simulink model "PotHoleHDLDetector"  (R2022a)
settings: Solver=FixedStepDiscrete  StartTime=0.0  StopTime=9  RelTol=1e-3
PreLoadFcn:
  | % Straight lines between these corners left,right and top,bottom
  | %        ltc---rtc
  | %        /       \
  | %       /         \
  | %      /           \
  | %   lbc-------------rbc
  | %
  | % For the 320x180 image:
  | raster = [320,180];
  | ltc = [155, 66];
  | lbc = [  1,140];
  | rtc = [155, 66];
  | rbc = [285,179];
  | 
  | % fit to x = f(y) for convienence
  | abl = polyfit([lbc(2),ltc(2)],[lbc(1),ltc(1)],1);  % left side
  | abr = polyfit([rbc(2),rtc(2)],[rbc(1),rtc(1)],1);  % right side
  | leftxstart = max(  1, round((ltc(2):rbc(2))*abl(1)+abl(2)));
  | rightxend  = min(raster(1), round((ltc(2):rbc(2))*abr(1)+abr(2)));
  | startline  = min(ltc(2),rtc(2));
  | endline    = max(lbc(2),rbc(2));
  | % correct values to zero-based
  | leftxstart = leftxstart - 1;
  | rightxend = rightxend - 1;
  | startline = startline - 1;
  | endline = endline - 1;
  | %%%%%%%%%%%%%%%%
  | % Character ROM for OSD
  | load charROM16x16.mat
  | %%%%%%%%%%%%%%%%
  | % Fiducial Marker (square reticle)
  | load fiducialROM31x31.mat
undefined symbols (not defined in the file or in its folder): charROM16x16, fiducialROM, gray, Rec, SDTV
libraries: hdlsllib x62, simulink x18, visionhdlutilities x7, visionhdlio x2, dspvision x1, visionhdlfilter x1, visionhdlmorphops x1, visionhdlconversions x1, visionhdlanalysis x1
(part 1 of 2)
settings Model: DataTypeOverride=Off  SimulationMode=accelerator  Creator=The MathWorks, Inc.  LastModifiedBy=ragha
settings SolverCC: AlgebraicLoopSolver=TrustRegion
settings DataIOCC: SaveOutput=off  SaveTime=off  ReturnWorkspaceOutputs=off
settings OptimizationCC: BlockReduction=off  ConditionallyExecuteInputs=off  DefaultParameterBehavior=Inlined  EfficientMapNaN2IntZero=off
settings DebuggingCC: AlgebraicLoopMsg=error  SingleTaskRateTransMsg=error  IntegerOverflowMsg=none  ParameterPrecisionLossMsg=none  UnconnectedInputMsg=warning  UnconnectedOutputMsg=warning  UnconnectedLineMsg=warning  SFMachineParentedDataDiag=warning  IntegerSaturationMsg=none  ArithmeticOperatorsInVariantConditions=warning
settings HardwareCC: ProdBitPerPointer=32  ProdBitPerSizeT=32  ProdBitPerPtrDiffT=32  ProdLargestAtomicFloat=None  ProdIntDivRoundTo=Undefined  ProdEndianess=Unspecified  ProdWordSize=32  ProdHWDeviceType=ASIC/FPGA->ASIC/FPGA  TargetBitPerPointer=64  TargetBitPerSizeT=64  TargetBitPerPtrDiffT=64  TargetLongLongMode=on  TargetIntDivRoundTo=Zero  TargetEndianess=LittleEndian  TargetWordSize=64  TargetHWDeviceType=MATLAB Host  ProdEqTarget=off
settings SFSimCC: SimUseLocalCustomCode=off
settings RTWCC: RTWUseLocalCustomCode=off  DLArmComputeVersion=19.05
settings CodeAppCC: MaxIdLength=128
settings GRTTargetCC: TargetLangStandard=C89/C90 (ANSI)  CombineOutputUpdateFcns=off  GRTInterface=on

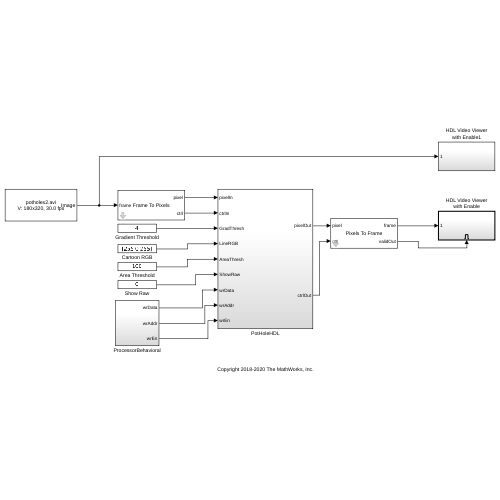
[thumbnail: Simulink's stored preview of the top-level diagram]
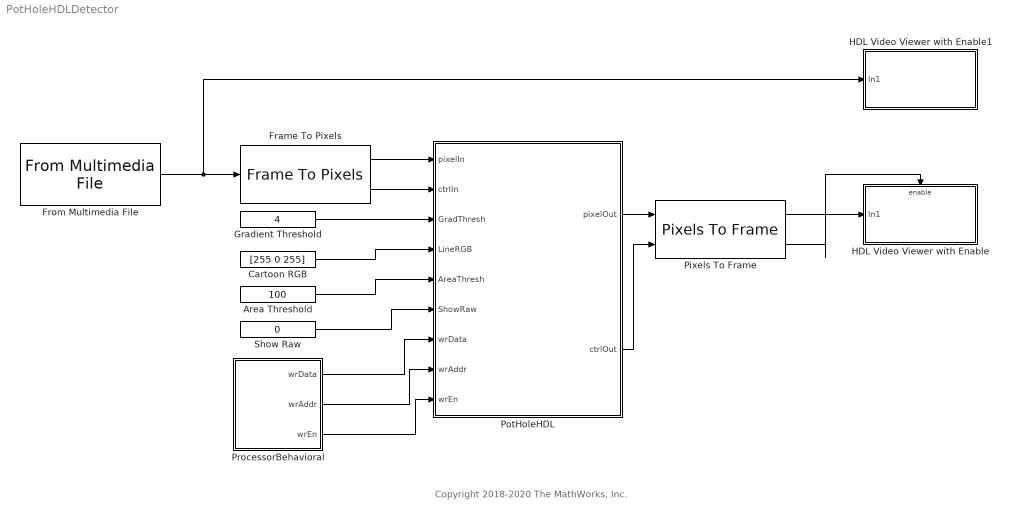
== system PotHoleHDLDetector ==
  note: Copyright 2018-2020 The MathWorks, Inc.
  "Area Threshold " : Constant  Value=100  OutDataTypeStr=fixdt(0,10,0)  SampleTime=-1
  Cartoon RGB : Constant  Value=[255 0 255]  OutDataTypeStr=uint8  SampleTime=-1
  Frame To Pixels : visionhdlio/Frame To Pixels  NumComponents=3  NumPixels=1  VideoFormat=Custom  ActivePixelsPerLine=320  ActiveVideoLines=180  TotalPixelsPerLine=400  TotalVideoLines=240  StartingActiveLine=6  FrontPorch=10  SampleTime=0  VideoFormatCache=Custom  ActivePixelsPerLineCache=320  ActiveVideoLinesCache=180  TotalPixelsPerLineCache=400  TotalVideoLinesCache=240  StartingActiveLineCache=6  FrontPorchCache=10
      settings: SourceProductBaseCode=VT
  From Multimedia File : dspvision/From Multimedia File  inputFilename=potholes2.avi  readRange=[1 Inf]  loop=on  numPlays=inf  outputStreams=Video only  videoDataType=uint8  audioDataType=int16  inheritSampleTime=on  userDefinedSampleTime=1/30  noAudioOutput=off  isIntensityVideo=off  fourcc=RGB  colorVideoFormat=One multidimensional signal  outputEOF=off  dataOrg=Column-major  audioFrameSize=1024  computeAudioFrameSize=off  outSamplingMode=Sample based
  Gradient Threshold : Constant  Value=4  OutDataTypeStr=uint8  SampleTime=-1
  HDL Video Viewer with Enable : Subsystem
  HDL Video Viewer with Enable1 : Subsystem
  Pixels To Frame : visionhdlio/Pixels To Frame  NumComponents=3  NumPixels=1  VideoFormat=Custom  ActivePixelsPerLine=320  ActiveVideoLines=180  TotalPixelsPerLine=400  TotalVideoLines=240  VideoFormatCache=Custom  ActivePixelsPerLineCache=320  ActiveVideoLinesCache=180  TotalPixelsPerLineCache=400  TotalVideoLinesCache=240
      settings: SourceProductBaseCode=VT
  PotHoleHDL : Subsystem
  ProcessorBehavioral : Subsystem
  Show Raw : Constant  Value=0  OutDataTypeStr=boolean  SampleTime=-1
  wires:
  Gradient Threshold/1 -> PotHoleHDL/3(GradThresh)
  Pixels To Frame/2 -> HDL Video Viewer with Enable/Enable
  Pixels To Frame/1 -> HDL Video Viewer with Enable/1(In1)
  PotHoleHDL/1(pixelOut) -> Pixels To Frame/1
  From Multimedia File/1 -> HDL Video Viewer with Enable1/1(In1), Frame To Pixels/1
  Cartoon RGB/1 -> PotHoleHDL/4(LineRGB)
  Frame To Pixels/2 -> PotHoleHDL/2(ctrlIn)
  Frame To Pixels/1 -> PotHoleHDL/1(pixelIn)
  "Area Threshold "/1 -> PotHoleHDL/5(AreaThresh)
  ProcessorBehavioral/1(wrData) -> PotHoleHDL/7("wrData ")
  ProcessorBehavioral/2(wrAddr) -> PotHoleHDL/8(wrAddr)
  ProcessorBehavioral/3(wrEn) -> PotHoleHDL/9(wrEn)
  Show Raw/1 -> PotHoleHDL/6(ShowRaw)
  PotHoleHDL/2(ctrlOut) -> Pixels To Frame/2

== system PotHoleHDLDetector/HDL Video Viewer with Enable ==
  In1 : Inport
  Enable : EnablePort
  PotHoleDisplay : VideoViewer  colormapValue=gray(256)  FigPos=[1 670 1280 574.666666666667]
  wires:
  In1/1 -> PotHoleDisplay/1

== system PotHoleHDLDetector/HDL Video Viewer with Enable1 ==
  In1 : Inport
  ImageIn : VideoViewer  colormapValue=gray(256)  FigPos=[128 352 321 244]
  wires:
  In1/1 -> ImageIn/1

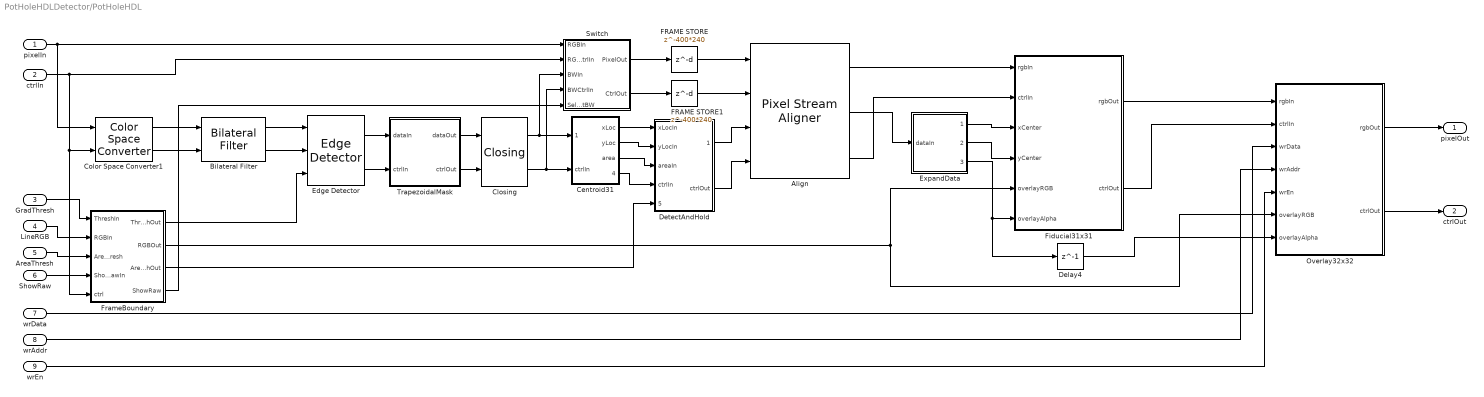
== system PotHoleHDLDetector/PotHoleHDL ==
  pixelIn : Inport
  ctrlIn : Inport  Port=2
  GradThresh : Inport  Port=3
  LineRGB : Inport  Port=4
  AreaThresh : Inport  Port=5
  ShowRaw : Inport  Port=6
  "wrData " : Inport  Port=7
  wrAddr : Inport  Port=8
  wrEn : Inport  Port=9
  Align : visionhdlutilities/Pixel Stream Aligner  LineBufferSize=2048  MaximumNumberOfLines=40  SimulateUsing=Code generation
      settings: SourceProductBaseCode=VT
  Bilateral Filter : visionhdlfilter/Bilateral Filter  NeighborhoodSize=9x9  SpatialStdDev=3  IntensityStdDev=0.75  PaddingMethod=Replicate  PaddingValue=0  LineBufferSize=2048  SimulateUsing=Code generation  CoefficientsDataTypeStr=fixdt(0,22,22)  roundingMode=Nearest  overflowMode=on  OutputDataTypeStr=fixdt(0,8,0)  OutputMin=[]  OutputMax=[]
      settings: SourceProductBaseCode=VT
  Centroid31 : Subsystem
  Closing : visionhdlmorphops/Closing  Neighborhood=[0 1 1 1 0;1 1 1 1 1;1 1 1 1 1;1 1 1 1 1;0 1 1 1 0]  LineBufferSize=2048  PaddingMethod=Constant  SimulateUsing=Code generation
      settings: SourceProductBaseCode=VT
  Color Space Converter1 : visionhdlconversions/Color Space Converter  Conversion=RGB to intensity  ConversionStandard=Rec. 601 (SDTV)  ScanningStandard=1250/50/2:1  SimulateUsing=Code generation
      settings: SourceProductBaseCode=VT
  Delay4 : Delay  DelayLength=1
  DetectAndHold : Subsystem
  Edge Detector : visionhdlanalysis/Edge Detector  Method=Sobel  BinaryImageOutputPort=on  GradientComponentOutputPorts=off  ThresholdSource=Input port  Threshold=20  LineBufferSize=2048  PaddingMethod=Symmetric  SimulateUsing=Code generation  roundingMode=Floor  overflowMode=off  GradientMin=[]  GradientMax=[]
      settings: SourceProductBaseCode=VT
  ExpandData : Subsystem
  FRAME STORE : Delay  DelayLength=400*240
  FRAME STORE1 : Delay  DelayLength=400*240
  Fiducial31x31 : Subsystem
  FrameBoundary : Subsystem
  Overlay32x32 : Subsystem
  Switch : Subsystem
  TrapezoidalMask : Subsystem
  pixelOut : Outport  VectorParamsAs1DForOutWhenUnconnected=off
  ctrlOut : Outport  Port=2  VectorParamsAs1DForOutWhenUnconnected=off
  wires:
  ctrlIn/1 -> FrameBoundary/5(ctrl), Color Space Converter1/2, Switch/2(RGBCtrlIn)
  pixelIn/1 -> Color Space Converter1/1, Switch/1(RGBIn)
  GradThresh/1 -> FrameBoundary/1(ThreshIn)
  LineRGB/1 -> FrameBoundary/2(RGBIn)
  FrameBoundary/1(ThreshOut) -> Edge Detector/3
  FrameBoundary/2(RGBOut) -> Fiducial31x31/5(overlayRGB), Overlay32x32/6(overlayRGB)
  wrEn/1 -> Overlay32x32/5(wrEn)
  Delay4/1 -> Overlay32x32/7(overlayAlpha)
  wrAddr/1 -> Overlay32x32/4(wrAddr)
  "wrData "/1 -> Overlay32x32/3(wrData)
  Overlay32x32/1(rgbOut) -> pixelOut/1
  Overlay32x32/2(ctrlOut) -> ctrlOut/1
  Closing/2 -> Switch/4(BWCtrlIn), Centroid31/2(ctrlIn)
  Color Space Converter1/1 -> Bilateral Filter/1
  Color Space Converter1/2 -> Bilateral Filter/2
  Bilateral Filter/1 -> Edge Detector/1
  Bilateral Filter/2 -> Edge Detector/2
  Edge Detector/1 -> TrapezoidalMask/1(dataIn)
  Edge Detector/2 -> TrapezoidalMask/2(ctrlIn)
  TrapezoidalMask/1(dataOut) -> Closing/1
  TrapezoidalMask/2(ctrlOut) -> Closing/2
  Closing/1 -> Switch/3(BWIn), Centroid31/1(pixelIn)
  Align/3 -> Fiducial31x31/2(ctrlIn)
  Align/1 -> Fiducial31x31/1(rgbIn)
  Fiducial31x31/2(ctrlOut) -> Overlay32x32/2(ctrlIn)
  Fiducial31x31/1(rgbOut) -> Overlay32x32/1(rgbIn)
  AreaThresh/1 -> FrameBoundary/3(AreaThresh)
  Centroid31/1(xLoc) -> DetectAndHold/1(xLocIn)
  Centroid31/2(yLoc) -> DetectAndHold/2(yLocIn)
  Centroid31/3(area) -> DetectAndHold/3(areaIn)
  FrameBoundary/3(AreaThreshOut) -> DetectAndHold/5(areaThresh)
  DetectAndHold/1(dataOut) -> Align/3
  Centroid31/4(ctrlOut) -> DetectAndHold/4(ctrlIn)
  DetectAndHold/2(ctrlOut) -> Align/4
  Align/2 -> ExpandData/1(dataIn)
  ExpandData/1(xLocOut) -> Fiducial31x31/3(xCenter)
  ExpandData/2(yLocOut) -> Fiducial31x31/4(yCenter)
  ExpandData/3(DetectOut) -> Delay4/1, Fiducial31x31/6(overlayAlpha)
  FRAME STORE/1 -> Align/1
  FRAME STORE1/1 -> Align/2
  ShowRaw/1 -> FrameBoundary/4(ShowRawIn)
  FrameBoundary/4(ShowRaw) -> Switch/5(SelectBW)
  Switch/1(PixelOut) -> FRAME STORE/1
  Switch/2(CtrlOut) -> FRAME STORE1/1

== system PotHoleHDLDetector/ProcessorBehavioral ==
  Bit Concat2 : hdlsllib/Logic and Bit Operations/Bit Concat  numInputs=2
  Constant3 : Constant  Value="uint8('     Pothole!');"
  Constant4 : Constant  Value=logical(0)
  Constant5 : Constant  Value=fi(0,0,3,0)
  Constant6 : Constant  Value=fi(0,0,2,0)
  HDL Counter2 : hdlsllib/Sources/HDL Counter  CountType=Count limited  CountInit=0  CountStep=1  CountMax=12  CountFromType=Initial value  CountFrom=0  CountResetPort=off  CountLoadPort=off  CountEnbPort=on  CountDirPort=off  CountHitOutputPort=off  CountDataType=Unsigned  CountWordLen=8  CountFracLen=0  CountSampTime=1
  Index Vector : MultiPortSwitch  DataPortOrder=Zero-based contiguous  Inputs=1  zeroidx=on  SaturateOnIntegerOverflow=off  InputSameDT=off
  Index Vector2 : MultiPortSwitch  DataPortOrder=Zero-based contiguous  Inputs=1  zeroidx=on  SaturateOnIntegerOverflow=off  InputSameDT=off
  Tapped Delay : simulink/Discrete/Tapped Delay  vinit=1  samptime=-1  NumDelays=13  DelayOrder=Oldest  includeCurrent=off
  wrData : Outport  VectorParamsAs1DForOutWhenUnconnected=off
  wrAddr : Outport  Port=2  VectorParamsAs1DForOutWhenUnconnected=off
  wrEn : Outport  Port=3  VectorParamsAs1DForOutWhenUnconnected=off
  wires:
  Tapped Delay/1 -> Index Vector/2
  Index Vector/1 -> wrEn/1, HDL Counter2/1
  Constant4/1 -> Tapped Delay/1
  Constant3/1 -> Index Vector2/2
  Index Vector2/1 -> wrData/1
  Constant6/1 -> Bit Concat2/1
  HDL Counter2/1 -> Bit Concat2/2, Index Vector2/1
  Constant5/1 -> Index Vector/1
  Bit Concat2/1 -> wrAddr/1

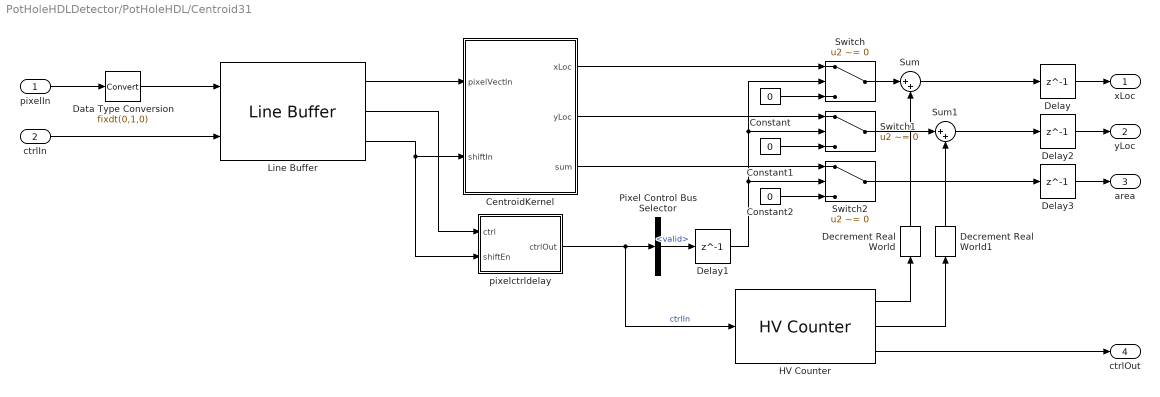
== system PotHoleHDLDetector/PotHoleHDL/Centroid31 ==
  pixelIn : Inport
  ctrlIn : Inport  Port=2
  CentroidKernel : Subsystem
  Constant : Constant  Value=0  OutDataTypeStr=Inherit: Inherit via back propagation
  Constant1 : Constant  Value=0  OutDataTypeStr=Inherit: Inherit via back propagation
  Constant2 : Constant  Value=0  OutDataTypeStr=Inherit: Inherit via back propagation
  Data Type Conversion : DataTypeConversion  OutDataTypeStr=fixdt(0,1,0)  SaturateOnIntegerOverflow=off  RndMeth=Floor
  Decrement Real World : simulink/Additional Math & Discrete/Additional Math: Increment - Decrement/Decrement Real World
      settings: SourceProductBaseCode=SL
  Decrement Real World1 : simulink/Additional Math & Discrete/Additional Math: Increment - Decrement/Decrement Real World
      settings: SourceProductBaseCode=SL
  Delay{,1..3} (4 alike) : Delay  DelayLength=1
  HV Counter : visionhdlutilities/HV Counter  ActivePixelsPerLine=320  ActiveVideoLines=180  SimulateUsing=Code generation
      settings: SourceProductBaseCode=VT
  Line Buffer : visionhdlutilities/Line Buffer  NeighborhoodSize=[31 31]  PaddingMethod=Constant  PaddingValue=0  LineBufferSize=2048  SimulateUsing=Code generation
      settings: SourceProductBaseCode=VT
  Pixel Control Bus Selector : BusSelector  OutputSignals=valid
  Sum : Sum  Inputs=|++  OutDataTypeStr=fixdt(0,11,0)  RndMeth=Convergent
  Sum1 : Sum  Inputs=|++  OutDataTypeStr=fixdt(0,11,0)  RndMeth=Convergent
  Switch : Switch  Criteria=u2 ~= 0  SaturateOnIntegerOverflow=off  InputSameDT=off
  Switch1 : Switch  Criteria=u2 ~= 0  SaturateOnIntegerOverflow=off  InputSameDT=off
  Switch2 : Switch  Criteria=u2 ~= 0  SaturateOnIntegerOverflow=off  InputSameDT=off
  pixelctrldelay : Subsystem
  xLoc : Outport  VectorParamsAs1DForOutWhenUnconnected=off
  yLoc : Outport  Port=2  VectorParamsAs1DForOutWhenUnconnected=off
  area : Outport  Port=3  VectorParamsAs1DForOutWhenUnconnected=off
  ctrlOut : Outport  Port=4  VectorParamsAs1DForOutWhenUnconnected=off
  wires:
  pixelIn/1 -> Data Type Conversion/1
  ctrlIn/1 -> Line Buffer/2
  Line Buffer/1 -> CentroidKernel/1(pixelVectIn)
  Line Buffer/3 -> pixelctrldelay/2(shiftEn), CentroidKernel/2(shiftIn)
  Data Type Conversion/1 -> Line Buffer/1
  pixelctrldelay/1(ctrlOut) -> HV Counter/1, Pixel Control Bus Selector/1  "ctrlIn"
  CentroidKernel/1(xLoc) -> Switch/1
  Switch2/1 -> Delay3/1
  CentroidKernel/2(yLoc) -> Switch1/1
  CentroidKernel/3(sum) -> Switch2/1
  Constant/1 -> Switch/3
  Constant1/1 -> Switch1/3
  Constant2/1 -> Switch2/3
  Pixel Control Bus Selector/1 -> Delay1/1  "<valid>"
  Delay/1 -> xLoc/1
  Delay2/1 -> yLoc/1
  Delay3/1 -> area/1
  Switch/1 -> Sum/1
  Sum/1 -> Delay/1
  Switch1/1 -> Sum1/1
  Sum1/1 -> Delay2/1
  Line Buffer/2 -> pixelctrldelay/1(ctrl)
  HV Counter/1 -> Decrement Real World/1
  HV Counter/2 -> Decrement Real World1/1
  HV Counter/3 -> ctrlOut/1
  Delay1/1 -> Switch2/2, Switch1/2, Switch/2
  Decrement Real World/1 -> Sum/2
  Decrement Real World1/1 -> Sum1/2

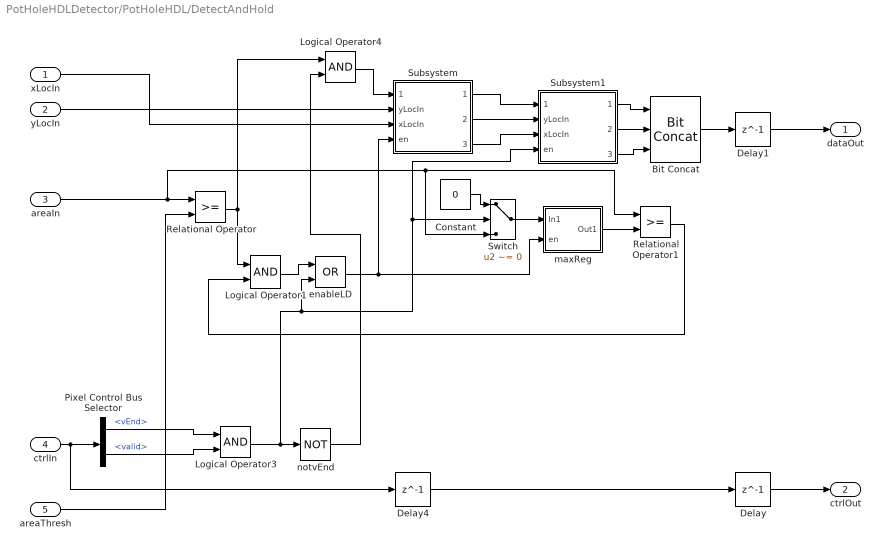
== system PotHoleHDLDetector/PotHoleHDL/DetectAndHold ==
  xLocIn : Inport
  yLocIn : Inport  Port=2
  areaIn : Inport  Port=3
  ctrlIn : Inport  Port=4
  areaThresh : Inport  Port=5
  Bit Concat : hdlsllib/Logic and Bit Operations/Bit Concat  numInputs=3
  Constant : Constant  Value=0  OutDataTypeStr=fixdt(0,10,0)
  Delay : Delay  DelayLength=1
  Delay1 : Delay  DelayLength=1
  Delay4 : Delay  DelayLength=1
  Logical Operator1 : Logic  AllPortsSameDT=off  OutDataTypeStr=boolean
  Logical Operator3 : Logic  AllPortsSameDT=off  OutDataTypeStr=boolean
  Logical Operator4 : Logic  AllPortsSameDT=off  OutDataTypeStr=boolean
  Pixel Control Bus Selector : BusSelector  OutputSignals=vEnd,valid
  Relational Operator : RelationalOperator  OutDataTypeStr=boolean  RndMeth=Simplest  InputSameDT=off
  Relational Operator1 : RelationalOperator  OutDataTypeStr=boolean  RndMeth=Simplest  InputSameDT=off
  Subsystem : Subsystem
  Subsystem1 : Subsystem
  Switch : Switch  Criteria=u2 ~= 0  SaturateOnIntegerOverflow=off  InputSameDT=off
  enableLD : Logic  Operator=OR  AllPortsSameDT=off  OutDataTypeStr=boolean
  maxReg : Subsystem
  notvEnd : Logic  Operator=NOT  AllPortsSameDT=off  OutDataTypeStr=boolean
  dataOut : Outport  VectorParamsAs1DForOutWhenUnconnected=off
  ctrlOut : Outport  Port=2  VectorParamsAs1DForOutWhenUnconnected=off
  wires:
  Logical Operator3/1 -> notvEnd/1, Subsystem1/4(en), Switch/2, enableLD/2
  areaIn/1 -> Switch/3, Relational Operator1/1, Relational Operator/1
  Pixel Control Bus Selector/1 -> Logical Operator3/1  "<vEnd>"
  Pixel Control Bus Selector/2 -> Logical Operator3/2  "<valid>"
  Relational Operator/1 -> Logical Operator4/1, Logical Operator1/1
  notvEnd/1 -> Logical Operator4/2
  ctrlIn/1 -> Pixel Control Bus Selector/1, Delay4/1
  areaThresh/1 -> Relational Operator/2
  Delay4/1 -> Delay/1
  Delay/1 -> ctrlOut/1
  Delay1/1 -> dataOut/1
  Logical Operator1/1 -> enableLD/1
  Logical Operator4/1 -> Subsystem/1(detectIn)
  maxReg/1(Out1) -> Relational Operator1/2
  enableLD/1 -> maxReg/2(en), Subsystem/4(en)
  Switch/1 -> maxReg/1(In1)
  Relational Operator1/1 -> Logical Operator1/2
  yLocIn/1 -> Subsystem/2(yLocIn)
  xLocIn/1 -> Subsystem/3(xLocIn)
  Subsystem/3(xLocOut) -> Subsystem1/3(xLocIn)
  Subsystem/2(yLocOut) -> Subsystem1/2(yLocIn)
  Subsystem/1(detectOut) -> Subsystem1/1(detectIn)
  Constant/1 -> Switch/1
  Subsystem1/2(yLocOut) -> Bit Concat/2
  Subsystem1/3(xLocOut) -> Bit Concat/3
  Subsystem1/1(detectOut) -> Bit Concat/1
  Bit Concat/1 -> Delay1/1

== system PotHoleHDLDetector/PotHoleHDL/ExpandData ==
  dataIn : Inport
  Bit Slice : hdlsllib/Logic and Bit Operations/Bit Slice  lidx=10  ridx=0
      settings: SourceProductBaseCode=SL
  Bit Slice1 : hdlsllib/Logic and Bit Operations/Bit Slice  lidx=21  ridx=11
      settings: SourceProductBaseCode=SL
  Bit Slice2 : hdlsllib/Logic and Bit Operations/Bit Slice  lidx=22  ridx=22
      settings: SourceProductBaseCode=SL
  Gain : Gain  Gain=255  ParamDataTypeStr=uint8  OutDataTypeStr=uint8
  xLocOut : Outport  VectorParamsAs1DForOutWhenUnconnected=off
  yLocOut : Outport  Port=2  VectorParamsAs1DForOutWhenUnconnected=off
  DetectOut : Outport  Port=3  VectorParamsAs1DForOutWhenUnconnected=off
  wires:
  Bit Slice2/1 -> Gain/1
  dataIn/1 -> Bit Slice2/1, Bit Slice1/1, Bit Slice/1
  Bit Slice/1 -> xLocOut/1
  Bit Slice1/1 -> yLocOut/1
  Gain/1 -> DetectOut/1

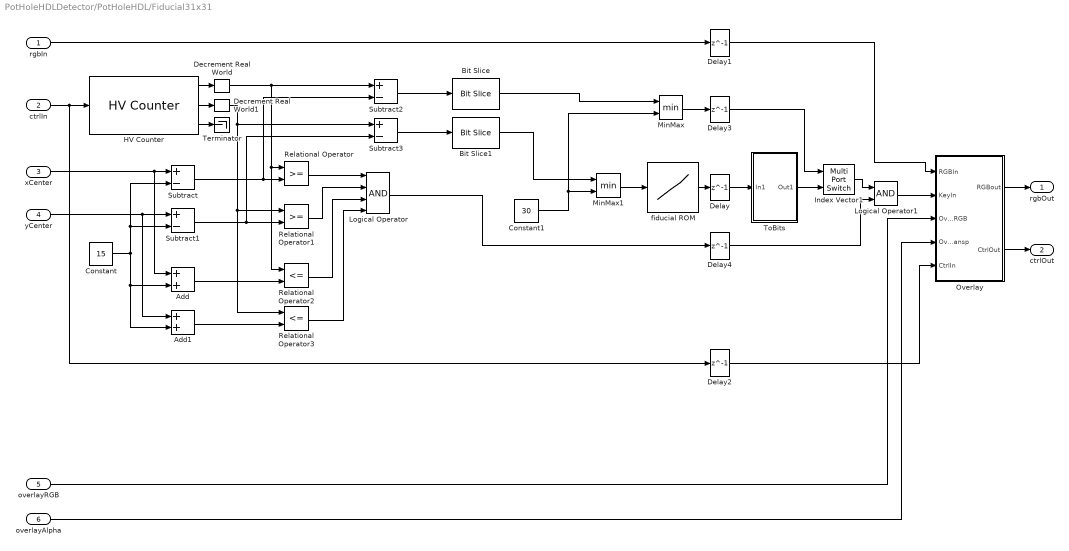
== system PotHoleHDLDetector/PotHoleHDL/Fiducial31x31 ==
  rgbIn : Inport
  ctrlIn : Inport  Port=2
  xCenter : Inport  Port=3
  yCenter : Inport  Port=4
  overlayRGB : Inport  Port=5
  overlayAlpha : Inport  Port=6
  Add : Sum
  Add1 : Sum
  Bit Slice : hdlsllib/Logic and Bit Operations/Bit Slice  lidx=4  ridx=0
      settings: SourceProductBaseCode=SL
  Bit Slice1 : hdlsllib/Logic and Bit Operations/Bit Slice  lidx=4  ridx=0
      settings: SourceProductBaseCode=SL
  Constant : Constant  Value=15  OutDataTypeStr=fixdt(0,11,0)
  Constant1 : Constant  Value=30  OutDataTypeStr=fixdt(0,5,0)
  Decrement Real World : simulink/Additional Math & Discrete/Additional Math: Increment - Decrement/Decrement Real World
      settings: SourceProductBaseCode=SL
  Decrement Real World1 : simulink/Additional Math & Discrete/Additional Math: Increment - Decrement/Decrement Real World
      settings: SourceProductBaseCode=SL
  Delay{,1..4} (5 alike) : Delay  DelayLength=1
  HV Counter : visionhdlutilities/HV Counter  ActivePixelsPerLine=1920  ActiveVideoLines=1080  SimulateUsing=Code generation
      settings: SourceProductBaseCode=VT
  Index Vector1 : MultiPortSwitch  DataPortOrder=Zero-based contiguous  Inputs=1  zeroidx=on  SaturateOnIntegerOverflow=off  InputSameDT=off
  Logical Operator : Logic  Inputs=4  AllPortsSameDT=off  OutDataTypeStr=boolean
  Logical Operator1 : Logic  AllPortsSameDT=off  OutDataTypeStr=boolean
  MinMax : MinMax  Inputs=2
  MinMax1 : MinMax  Inputs=2
  Overlay : Subsystem
  Relational Operator : RelationalOperator  OutDataTypeStr=boolean  RndMeth=Simplest  InputSameDT=off
  Relational Operator1 : RelationalOperator  OutDataTypeStr=boolean  RndMeth=Simplest  InputSameDT=off
  Relational Operator2 : RelationalOperator  Operator=<=  OutDataTypeStr=boolean  RndMeth=Simplest  InputSameDT=off
  Relational Operator3 : RelationalOperator  Operator=<=  OutDataTypeStr=boolean  RndMeth=Simplest  InputSameDT=off
  Subtract{,1..3} (4 alike) : Sum  Inputs=+-
  Terminator : Terminator
  ToBits : Subsystem
  fiducial ROM : Lookup_n-D  NumberOfTableDimensions=1  LookupTableObject=''  BreakpointsForDimension1=[0:30]  BreakpointsForDimension1FirstPoint=10  BreakpointsForDimension2FirstPoint=10  BreakpointsForDimension1Spacing=12  BreakpointsForDimension2Spacing=12  IndexSearchMethod=Evenly spaced points  Table=fiducialROM  TableDataTypeStr=fixdt(0,31,0)  InterpMethod=Flat  DiagnosticForOutOfRangeInput=Error  InternalRulePriority=Speed  OutDataTypeStr=fixdt(0,31,0)  RndMeth=Simplest
  rgbOut : Outport  VectorParamsAs1DForOutWhenUnconnected=off
  ctrlOut : Outport  Port=2  VectorParamsAs1DForOutWhenUnconnected=off
  wires:
  ctrlIn/1 -> Delay2/1, HV Counter/1
  rgbIn/1 -> Delay1/1
  Overlay/2("CtrlOut ") -> ctrlOut/1
  Decrement Real World/1 -> Relational Operator2/1, Relational Operator/1, Subtract2/1
  fiducial ROM/1 -> Delay/1
  overlayRGB/1 -> Overlay/3(OverlayRGB)
  overlayAlpha/1 -> Overlay/4(OverlayTransp)
  Delay2/1 -> Overlay/5(CtrlIn)
  Overlay/1(RGBout) -> rgbOut/1
  Delay1/1 -> Overlay/1(RGBIn)
  Delay3/1 -> Index Vector1/1
  Decrement Real World1/1 -> Subtract3/1, Relational Operator1/1, Relational Operator3/1
  xCenter/1 -> Add/1, Subtract/1
  yCenter/1 -> Add1/1, Subtract1/1
  Constant/1 -> Add/2, Add1/2, Subtract1/2, Subtract/2
  Subtract/1 -> Subtract2/2, Relational Operator/2
  Subtract1/1 -> Subtract3/2, Relational Operator1/2
  Add/1 -> Relational Operator2/2
  Add1/1 -> Relational Operator3/2
  Relational Operator/1 -> Logical Operator/1
  Relational Operator1/1 -> Logical Operator/2
  Relational Operator2/1 -> Logical Operator/3
  Relational Operator3/1 -> Logical Operator/4
  Logical Operator/1 -> Delay4/1
  Subtract2/1 -> Bit Slice/1
  Subtract3/1 -> Bit Slice1/1
  Index Vector1/1 -> Logical Operator1/1
  Delay4/1 -> Logical Operator1/2
  Bit Slice/1 -> MinMax/1
  MinMax/1 -> Delay3/1
  Constant1/1 -> MinMax1/2, MinMax/2
  MinMax1/1 -> fiducial ROM/1
  Bit Slice1/1 -> MinMax1/1
  Logical Operator1/1 -> Overlay/2(KeyIn)
  ToBits/1(Out1) -> Index Vector1/2
  Delay/1 -> ToBits/1(In1)
  HV Counter/1 -> Decrement Real World/1
  HV Counter/2 -> Decrement Real World1/1
  HV Counter/3 -> Terminator/1

== system PotHoleHDLDetector/PotHoleHDL/FrameBoundary ==
  ThreshIn : Inport
  RGBIn : Inport  Port=2
  AreaThresh : Inport  Port=3
  ShowRawIn : Inport  Port=4
  ctrl : Inport  Port=5
  Delay{,1..3} (4 alike) : Delay  DelayLength=1  ShowEnablePort=on
      settings: InputPortMap=u0,e6
  Logical Operator : Logic  AllPortsSameDT=off  OutDataTypeStr=boolean
  Pixel Control Bus Selector : BusSelector  OutputSignals=vStart,valid
  ThreshOut : Outport  VectorParamsAs1DForOutWhenUnconnected=off
  RGBOut : Outport  Port=2  VectorParamsAs1DForOutWhenUnconnected=off
  AreaThreshOut : Outport  Port=3  VectorParamsAs1DForOutWhenUnconnected=off
  ShowRaw : Outport  Port=4  VectorParamsAs1DForOutWhenUnconnected=off
  wires:
  ctrl/1 -> Pixel Control Bus Selector/1
  Pixel Control Bus Selector/1 -> Logical Operator/1  "<vStart>"
  ThreshIn/1 -> Delay/1
  Logical Operator/1 -> Delay3/2, Delay2/2, Delay1/2, Delay/2
  Pixel Control Bus Selector/2 -> Logical Operator/2  "<valid>"
  Delay1/1 -> RGBOut/1
  RGBIn/1 -> Delay1/1
  Delay/1 -> ThreshOut/1
  AreaThresh/1 -> Delay2/1
  Delay2/1 -> AreaThreshOut/1
  Delay3/1 -> ShowRaw/1
  ShowRawIn/1 -> Delay3/1

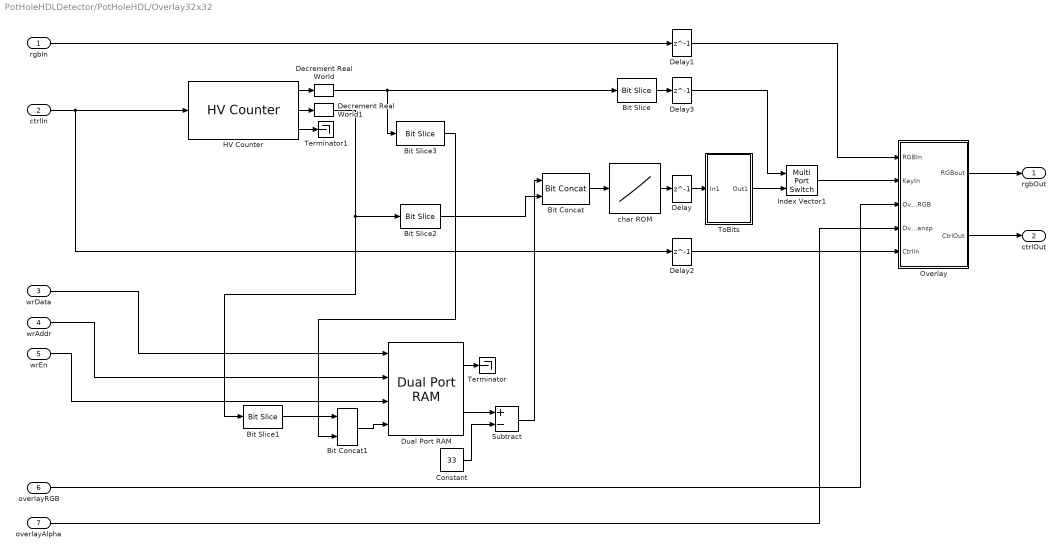
== system PotHoleHDLDetector/PotHoleHDL/Overlay32x32 ==
  rgbIn : Inport
  ctrlIn : Inport  Port=2
  wrData : Inport  Port=3
  wrAddr : Inport  Port=4
  wrEn : Inport  Port=5
  overlayRGB : Inport  Port=6
  overlayAlpha : Inport  Port=7
  Bit Concat : hdlsllib/Logic and Bit Operations/Bit Concat  numInputs=2
  Bit Concat1 : hdlsllib/Logic and Bit Operations/Bit Concat  numInputs=2
  Bit Slice : hdlsllib/Logic and Bit Operations/Bit Slice  lidx=3  ridx=0
      settings: SourceProductBaseCode=SL
  Bit Slice1 : hdlsllib/Logic and Bit Operations/Bit Slice  lidx=8  ridx=4
      settings: SourceProductBaseCode=SL
  Bit Slice2 : hdlsllib/Logic and Bit Operations/Bit Slice  lidx=3  ridx=0
      settings: SourceProductBaseCode=SL
  Bit Slice3 : hdlsllib/Logic and Bit Operations/Bit Slice  lidx=8  ridx=4
      settings: SourceProductBaseCode=SL
  Constant : Constant  Value=33  OutDataTypeStr=uint8
  Decrement Real World : simulink/Additional Math & Discrete/Additional Math: Increment - Decrement/Decrement Real World
      settings: SourceProductBaseCode=SL
  Decrement Real World1 : simulink/Additional Math & Discrete/Additional Math: Increment - Decrement/Decrement Real World
      settings: SourceProductBaseCode=SL
  Delay{,1..3} (4 alike) : Delay  DelayLength=1
  Dual Port RAM : hdlsllib/HDL RAMs/Dual Port RAM  ram_size=10
      settings: SourceProductBaseCode=SL
  HV Counter : visionhdlutilities/HV Counter  ActivePixelsPerLine=1920  ActiveVideoLines=1080  SimulateUsing=Code generation
      settings: SourceProductBaseCode=VT
  Index Vector1 : MultiPortSwitch  DataPortOrder=Zero-based contiguous  Inputs=1  zeroidx=on  SaturateOnIntegerOverflow=off  InputSameDT=off
  Overlay : Subsystem
  Subtract : Sum  Inputs=+-  OutDataTypeStr=fixdt(0,7,0)
  Terminator : Terminator
  Terminator1 : Terminator
  ToBits : Subsystem
  char ROM : Lookup_n-D  NumberOfTableDimensions=1  LookupTableObject=''  BreakpointsForDimension1=[0:128*16-1]  BreakpointsForDimension1FirstPoint=10  BreakpointsForDimension2FirstPoint=10  BreakpointsForDimension1Spacing=12  BreakpointsForDimension2Spacing=12  IndexSearchMethod=Evenly spaced points  Table=charROM16x16  TableDataTypeStr=fixdt(0,16,0)  InterpMethod=Flat  DiagnosticForOutOfRangeInput=Error  InternalRulePriority=Speed  OutDataTypeStr=fixdt(0,16,0)  RndMeth=Simplest
  rgbOut : Outport  VectorParamsAs1DForOutWhenUnconnected=off
  ctrlOut : Outport  Port=2  VectorParamsAs1DForOutWhenUnconnected=off
  wires:
  ctrlIn/1 -> Delay2/1, HV Counter/1
  rgbIn/1 -> Delay1/1
  Overlay/2("CtrlOut ") -> ctrlOut/1
  Bit Slice/1 -> Delay3/1
  ToBits/1(Out1) -> Index Vector1/2
  HV Counter/1 -> Decrement Real World/1
  Index Vector1/1 -> Overlay/2(KeyIn)
  Delay/1 -> ToBits/1(In1)
  Bit Concat/1 -> char ROM/1
  char ROM/1 -> Delay/1
  overlayRGB/1 -> Overlay/3(OverlayRGB)
  overlayAlpha/1 -> Overlay/4(OverlayTransp)
  Delay2/1 -> Overlay/5(CtrlIn)
  Overlay/1(RGBout) -> rgbOut/1
  Delay1/1 -> Overlay/1(RGBIn)
  Delay3/1 -> Index Vector1/1
  Bit Slice2/1 -> Bit Concat/2
  HV Counter/2 -> Decrement Real World1/1
  Subtract/1 -> Bit Concat/1
  Dual Port RAM/2 -> Subtract/1
  Constant/1 -> Subtract/2
  Bit Concat1/1 -> Dual Port RAM/4
  Bit Slice3/1 -> Bit Concat1/2
  Bit Slice1/1 -> Bit Concat1/1
  wrData/1 -> Dual Port RAM/1
  wrAddr/1 -> Dual Port RAM/2
  wrEn/1 -> Dual Port RAM/3
  Dual Port RAM/1 -> Terminator/1
  HV Counter/3 -> Terminator1/1
  Decrement Real World/1 -> Bit Slice3/1, Bit Slice/1
  Decrement Real World1/1 -> Bit Slice1/1, Bit Slice2/1

== system PotHoleHDLDetector/PotHoleHDL/Switch ==
  RGBIn : Inport
  RGBCtrlIn : Inport  Port=2
  BWIn : Inport  Port=3
  BWCtrlIn : Inport  Port=4
  SelectBW : Inport  Port=5
  Gain1 : Gain  Gain=255  ParamDataTypeStr=uint8  OutDataTypeStr=uint8
  Mux : Mux  Inputs=3
  Switch : Switch  Criteria=u2 ~= 0  SaturateOnIntegerOverflow=off  InputSameDT=off
  Switch1 : Switch  Criteria=u2 ~= 0  SaturateOnIntegerOverflow=off  InputSameDT=off
  PixelOut : Outport  VectorParamsAs1DForOutWhenUnconnected=off
  CtrlOut : Outport  Port=2  VectorParamsAs1DForOutWhenUnconnected=off
  wires:
  RGBCtrlIn/1 -> Switch1/3
  Gain1/1 -> Mux/3, Mux/2, Mux/1
  Mux/1 -> Switch/1
  Switch/1 -> PixelOut/1
  BWCtrlIn/1 -> Switch1/1
  SelectBW/1 -> Switch1/2, Switch/2
  RGBIn/1 -> Switch/3
  BWIn/1 -> Gain1/1
  Switch1/1 -> CtrlOut/1

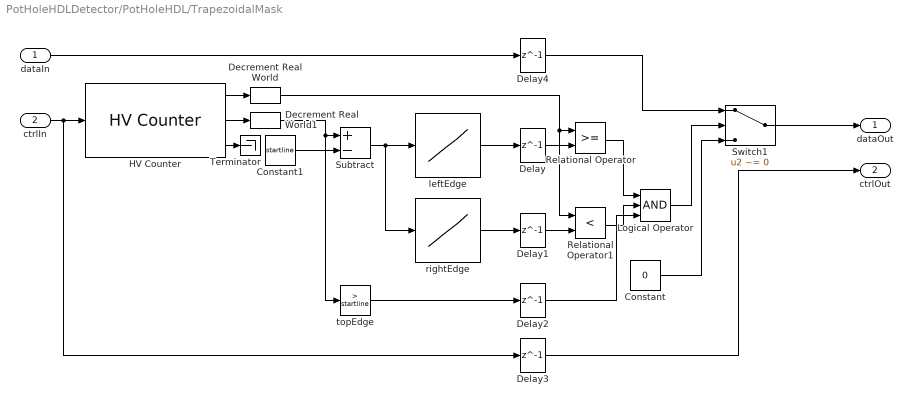
== system PotHoleHDLDetector/PotHoleHDL/TrapezoidalMask ==
  dataIn : Inport
  ctrlIn : Inport  Port=2
  Constant : Constant  Value=0  OutDataTypeStr=Inherit: Inherit via back propagation
  Constant1 : Constant  Value=startline  OutDataTypeStr=fixdt(0,11,0)
  Decrement Real World : simulink/Additional Math & Discrete/Additional Math: Increment - Decrement/Decrement Real World
      settings: SourceProductBaseCode=SL
  Decrement Real World1 : simulink/Additional Math & Discrete/Additional Math: Increment - Decrement/Decrement Real World
      settings: SourceProductBaseCode=SL
  Delay{,1..4} (5 alike) : Delay  DelayLength=1
  HV Counter : visionhdlutilities/HV Counter  ActivePixelsPerLine=320  ActiveVideoLines=240  SimulateUsing=Code generation
      settings: SourceProductBaseCode=VT
  Logical Operator : Logic  Inputs=3  AllPortsSameDT=off  OutDataTypeStr=boolean
  Relational Operator : RelationalOperator  OutDataTypeStr=boolean  RndMeth=Simplest  InputSameDT=off
  Relational Operator1 : RelationalOperator  Operator=<  OutDataTypeStr=boolean  RndMeth=Simplest  InputSameDT=off
  Subtract : Sum  Inputs=+-  OutDataTypeStr=Inherit: Same as first input
  Switch1 : Switch  Criteria=u2 ~= 0  SaturateOnIntegerOverflow=off  InputSameDT=off
  Terminator : Terminator
  leftEdge : Lookup_n-D  NumberOfTableDimensions=1  LookupTableObject=''  BreakpointsForDimension1=[0:113]  BreakpointsForDimension1FirstPoint=10  BreakpointsForDimension2FirstPoint=10  BreakpointsForDimension1Spacing=12  BreakpointsForDimension2Spacing=12  IndexSearchMethod=Evenly spaced points  Table=leftxstart  TableDataTypeStr=fixdt(0,11,0)  InterpMethod=Flat  InternalRulePriority=Speed  OutDataTypeStr=fixdt(0,11,0)  RndMeth=Simplest
  rightEdge : Lookup_n-D  NumberOfTableDimensions=1  LookupTableObject=''  BreakpointsForDimension1=[0:113]  BreakpointsForDimension1FirstPoint=10  BreakpointsForDimension2FirstPoint=10  BreakpointsForDimension1Spacing=12  BreakpointsForDimension2Spacing=12  IndexSearchMethod=Evenly spaced points  Table=rightxend  TableDataTypeStr=fixdt(0,11,0)  InterpMethod=Flat  InternalRulePriority=Speed  OutDataTypeStr=fixdt(0,11,0)  RndMeth=Simplest
  topEdge : simulink/Logic and Bit Operations/Compare To Constant  relop=>  const=startline  OutDataTypeStr=boolean
  dataOut : Outport  VectorParamsAs1DForOutWhenUnconnected=off
  ctrlOut : Outport  Port=2  VectorParamsAs1DForOutWhenUnconnected=off
  wires:
  rightEdge/1 -> Delay1/1
  topEdge/1 -> Delay2/1
  HV Counter/1 -> Decrement Real World/1
  leftEdge/1 -> Delay/1
  HV Counter/2 -> Decrement Real World1/1
  Relational Operator1/1 -> Logical Operator/2
  Logical Operator/1 -> Switch1/2
  Constant/1 -> Switch1/3
  Relational Operator/1 -> Logical Operator/1
  Delay2/1 -> Logical Operator/3
  Delay1/1 -> Relational Operator1/2
  Delay/1 -> Relational Operator/2
  dataIn/1 -> Delay4/1
  Switch1/1 -> dataOut/1
  ctrlIn/1 -> HV Counter/1, Delay3/1
  Delay3/1 -> ctrlOut/1
  Subtract/1 -> rightEdge/1, leftEdge/1
  Constant1/1 -> Subtract/2
  Delay4/1 -> Switch1/1
  HV Counter/3 -> Terminator/1
  Decrement Real World/1 -> Relational Operator1/1, Relational Operator/1
  Decrement Real World1/1 -> Subtract/1, topEdge/1

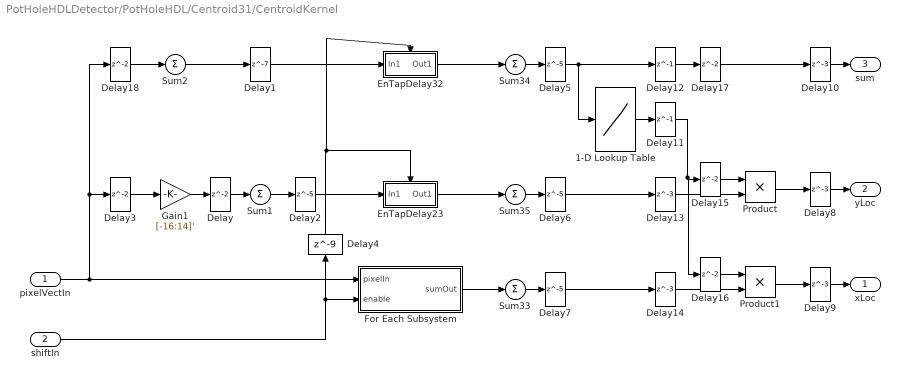
== system PotHoleHDLDetector/PotHoleHDL/Centroid31/CentroidKernel ==
  pixelVectIn : Inport
  shiftIn : Inport  Port=2
  1-D Lookup Table : Lookup_n-D  NumberOfTableDimensions=1  LookupTableObject=''  BreakpointsForDimension1=[0:1023]  BreakpointsForDimension1FirstPoint=10  BreakpointsForDimension2FirstPoint=10  BreakpointsForDimension1Spacing=12  BreakpointsForDimension2Spacing=12  IndexSearchMethod=Evenly spaced points  Table=1./[1,1:1023]  TableDataTypeStr=fixdt(0,15,15)  InterpMethod=Flat  DiagnosticForOutOfRangeInput=Error  InternalRulePriority=Speed  OutDataTypeStr=fixdt(0,15,15)  RndMeth=Simplest
  Delay{,3,15..18} (6 alike) : Delay
  Delay1 : Delay  DelayLength=7
  Delay{8..10,13..14} (5 alike) : Delay  DelayLength=3
  Delay11 : Delay  DelayLength=1
  Delay12 : Delay  DelayLength=1
  Delay{2,5..7} (4 alike) : Delay  DelayLength=5
  Delay4 : Delay  DelayLength=9
  EnTapDelay23 : Subsystem
  EnTapDelay32 : Subsystem
  For Each Subsystem : Subsystem  TreatAsAtomicUnit=on
  Gain1 : Gain  Gain=[-16:14]'  ParamDataTypeStr=fixdt(1,5,0)  OutDataTypeStr=fixdt(1,5,0)
  Product : Product  OutDataTypeStr=fixdt(1,8,3)  RndMeth=Nearest  SaturateOnIntegerOverflow=on
  Product1 : Product  OutDataTypeStr=fixdt(1,8,3)  RndMeth=Nearest  SaturateOnIntegerOverflow=on
  Sum{1..2,33..35} (5 alike) : Sum  Inputs=1
  xLoc : Outport  VectorParamsAs1DForOutWhenUnconnected=off
  yLoc : Outport  Port=2  VectorParamsAs1DForOutWhenUnconnected=off
  sum : Outport  Port=3  VectorParamsAs1DForOutWhenUnconnected=off
  wires:
  pixelVectIn/1 -> For Each Subsystem/1(pixelIn), Delay18/1, Delay3/1
  Sum1/1 -> Delay2/1
  EnTapDelay23/1(Out1) -> Sum35/1
  EnTapDelay32/1(Out1) -> Sum34/1
  Sum34/1 -> Delay5/1
  Product/1 -> Delay8/1
  Sum35/1 -> Delay6/1
  Product1/1 -> Delay9/1
  Sum33/1 -> Delay7/1
  1-D Lookup Table/1 -> Delay11/1
  shiftIn/1 -> For Each Subsystem/2(enable), Delay4/1
  For Each Subsystem/1(sumOut) -> Sum33/1
  Delay1/1 -> EnTapDelay32/1(In1)
  Delay2/1 -> EnTapDelay23/1(In1)
  Delay/1 -> Sum1/1
  Gain1/1 -> Delay/1
  Delay3/1 -> Gain1/1
  Delay4/1 -> EnTapDelay32/Enable, EnTapDelay23/Enable
  Delay5/1 -> 1-D Lookup Table/1, Delay12/1
  Delay6/1 -> Delay13/1
  Delay7/1 -> Delay14/1
  Delay8/1 -> yLoc/1
  Delay9/1 -> xLoc/1
  Delay10/1 -> sum/1
  Delay11/1 -> Delay16/1, Delay15/1
  Delay12/1 -> Delay17/1
  Delay13/1 -> Product/2
  Delay14/1 -> Product1/2
  Delay15/1 -> Product/1
  Delay16/1 -> Product1/1
  Delay17/1 -> Delay10/1
  Delay18/1 -> Sum2/1
  Sum2/1 -> Delay1/1

== system PotHoleHDLDetector/PotHoleHDL/Centroid31/pixelctrldelay ==
  ctrl : Inport
  shiftEn : Inport  Port=2
  Bitwise AND{,1..4} (5 alike) : simulink/Logic and Bit Operations/Bitwise Operator  logicop=AND  UseBitMask=off  NumInputPorts=2  BitMask=bin2dec('11011001')  BitMaskRealWorld=Stored Integer
  Delay : Delay  DelayLength=16  ShowEnablePort=on
      settings: InputPortMap=u0,e6
  Delay1 : Delay  DelayLength=1
  Delay2 : Delay  DelayLength=19
  Pixel Control Bus Creator : visionhdlutilities/Pixel Control Bus Creator
      settings: SourceProductBaseCode=VT
  Pixel Control Bus Selector : BusSelector  OutputSignals=hStart,hEnd,vStart,vEnd,valid
  State Control : StateControl  StateControl=Synchronous
  ctrlOut : Outport  VectorParamsAs1DForOutWhenUnconnected=off
  wires:
  Bitwise AND4/1 -> Pixel Control Bus Creator/5
  Bitwise AND/1 -> Pixel Control Bus Creator/1
  Pixel Control Bus Selector/3 -> Bitwise AND2/1  "<vStart>"
  Bitwise AND3/1 -> Pixel Control Bus Creator/4
  Pixel Control Bus Selector/5 -> Bitwise AND4/1  "<valid>"
  Delay/1 -> Pixel Control Bus Selector/1
  Pixel Control Bus Selector/1 -> Bitwise AND/1  "<hStart>"
  Pixel Control Bus Selector/2 -> Bitwise AND1/1  "<hEnd>"
  Bitwise AND2/1 -> Pixel Control Bus Creator/3
  Pixel Control Bus Selector/4 -> Bitwise AND3/1  "<vEnd>"
  Bitwise AND1/1 -> Pixel Control Bus Creator/2
  Pixel Control Bus Creator/1 -> Delay2/1
  ctrl/1 -> Delay/1
  shiftEn/1 -> Delay1/1, Delay/2
  Delay1/1 -> Bitwise AND3/2, Bitwise AND2/2, Bitwise AND1/2, Bitwise AND/2, Bitwise AND4/2
  Delay2/1 -> ctrlOut/1

== system PotHoleHDLDetector/PotHoleHDL/DetectAndHold/Subsystem ==
  detectIn : Inport
  yLocIn : Inport  Port=2
  xLocIn : Inport  Port=3
  en : Inport  Port=4
  Delay : Delay  DelayLength=1  ShowEnablePort=on
      settings: InputPortMap=u0,e6
  Delay1 : Delay  DelayLength=1  ShowEnablePort=on
      settings: InputPortMap=u0,e6
  Delay2 : Delay  DelayLength=1  ShowEnablePort=on
      settings: InputPortMap=u0,e6
  State Control : StateControl  StateControl=Synchronous
  detectOut : Outport  VectorParamsAs1DForOutWhenUnconnected=off
  yLocOut : Outport  Port=2  VectorParamsAs1DForOutWhenUnconnected=off
  xLocOut : Outport  Port=3  VectorParamsAs1DForOutWhenUnconnected=off
  wires:
  Delay1/1 -> xLocOut/1
  Delay/1 -> yLocOut/1
  Delay2/1 -> detectOut/1
  en/1 -> Delay1/2, Delay/2, Delay2/2
  xLocIn/1 -> Delay1/1
  yLocIn/1 -> Delay/1
  detectIn/1 -> Delay2/1

== system PotHoleHDLDetector/PotHoleHDL/DetectAndHold/Subsystem1 ==
  detectIn : Inport
  yLocIn : Inport  Port=2
  xLocIn : Inport  Port=3
  en : Inport  Port=4
  Delay : Delay  DelayLength=1  ShowEnablePort=on
      settings: InputPortMap=u0,e6
  Delay1 : Delay  DelayLength=1  ShowEnablePort=on
      settings: InputPortMap=u0,e6
  Delay2 : Delay  DelayLength=1  ShowEnablePort=on
      settings: InputPortMap=u0,e6
  State Control : StateControl  StateControl=Synchronous
  detectOut : Outport  VectorParamsAs1DForOutWhenUnconnected=off
  yLocOut : Outport  Port=2  VectorParamsAs1DForOutWhenUnconnected=off
  xLocOut : Outport  Port=3  VectorParamsAs1DForOutWhenUnconnected=off
  wires:
  detectIn/1 -> Delay2/1
  yLocIn/1 -> Delay/1
  xLocIn/1 -> Delay1/1
  en/1 -> Delay2/2, Delay/2, Delay1/2
  Delay2/1 -> detectOut/1
  Delay/1 -> yLocOut/1
  Delay1/1 -> xLocOut/1

== system PotHoleHDLDetector/PotHoleHDL/DetectAndHold/maxReg ==
  In1 : Inport
  en : Inport  Port=2
  Delay : Delay  DelayLength=1  ShowEnablePort=on
      settings: InputPortMap=u0,e6
  State Control : StateControl  StateControl=Synchronous
  Out1 : Outport  VectorParamsAs1DForOutWhenUnconnected=off
  wires:
  In1/1 -> Delay/1
  Delay/1 -> Out1/1
  en/1 -> Delay/2

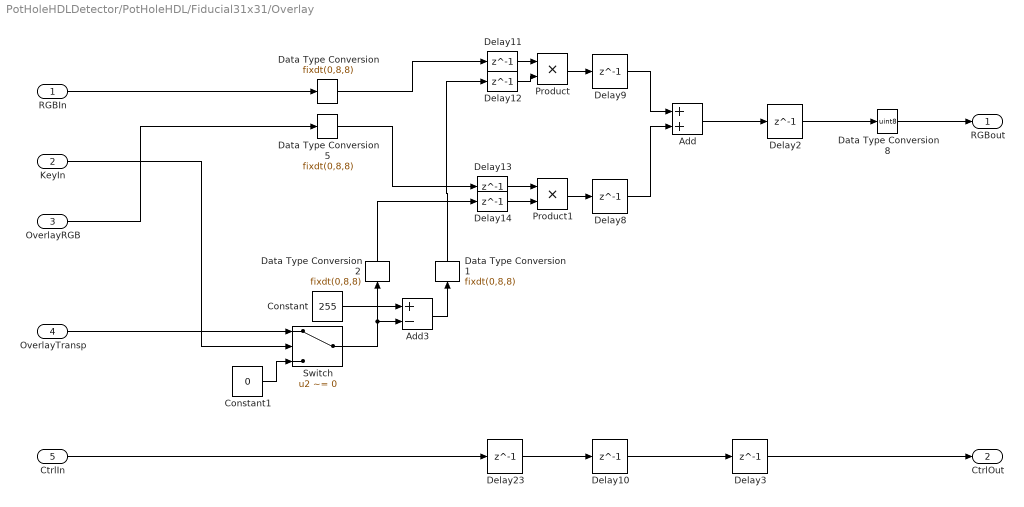
== system PotHoleHDLDetector/PotHoleHDL/Fiducial31x31/Overlay ==
  RGBIn : Inport
  KeyIn : Inport  Port=2
  OverlayRGB : Inport  Port=3
  OverlayTransp : Inport  Port=4
  CtrlIn : Inport  Port=5
  Add : Sum  OutDataTypeStr=fixdt(0,8,8)
  Add3 : Sum  Inputs=+-  OutDataTypeStr=uint8
  Constant : Constant  Value=255  OutDataTypeStr=uint8  SampleTime=-1
  Constant1 : Constant  Value=0  OutDataTypeStr=uint8
  Data Type Conversion{,1..2,5} (4 alike) : DataTypeConversion  OutDataTypeStr=fixdt(0,8,8)  ConvertRealWorld=Stored Integer (SI)  SaturateOnIntegerOverflow=off  RndMeth=Floor
  Data Type Conversion8 : DataTypeConversion  OutDataTypeStr=uint8  ConvertRealWorld=Stored Integer (SI)  SaturateOnIntegerOverflow=off  RndMeth=Floor
  Delay{2..3,8..14,23} (10 alike) : Delay  DelayLength=1
  Product : Product  OutDataTypeStr=fixdt(0,8,8)  SaturateOnIntegerOverflow=on
  Product1 : Product  OutDataTypeStr=fixdt(0,8,8)  SaturateOnIntegerOverflow=on
  Switch : Switch  Criteria=u2 ~= 0  SaturateOnIntegerOverflow=off  InputSameDT=off
  RGBout : Outport  VectorParamsAs1DForOutWhenUnconnected=off
  "CtrlOut " : Outport  Port=2  VectorParamsAs1DForOutWhenUnconnected=off
  wires:
  Add/1 -> Delay2/1
  Constant/1 -> Add3/1
  Add3/1 -> Data Type Conversion1/1
  Switch/1 -> Data Type Conversion2/1, Add3/2
  OverlayTransp/1 -> Switch/1
  KeyIn/1 -> Switch/2
  Constant1/1 -> Switch/3
  Delay2/1 -> Data Type Conversion8/1
  Delay3/1 -> "CtrlOut "/1
  Product1/1 -> Delay8/1
  Product/1 -> Delay9/1
  Delay9/1 -> Add/1
  Delay8/1 -> Add/2
  Delay10/1 -> Delay3/1
  Delay11/1 -> Product/1
  Delay12/1 -> Product/2
  Delay13/1 -> Product1/1
  Delay14/1 -> Product1/2
  Delay23/1 -> Delay10/1
  CtrlIn/1 -> Delay23/1
  Data Type Conversion/1 -> Delay11/1
  Data Type Conversion1/1 -> Delay12/1
  Data Type Conversion2/1 -> Delay14/1
  OverlayRGB/1 -> Data Type Conversion5/1
  RGBIn/1 -> Data Type Conversion/1
  Data Type Conversion8/1 -> RGBout/1
  Data Type Conversion5/1 -> Delay13/1

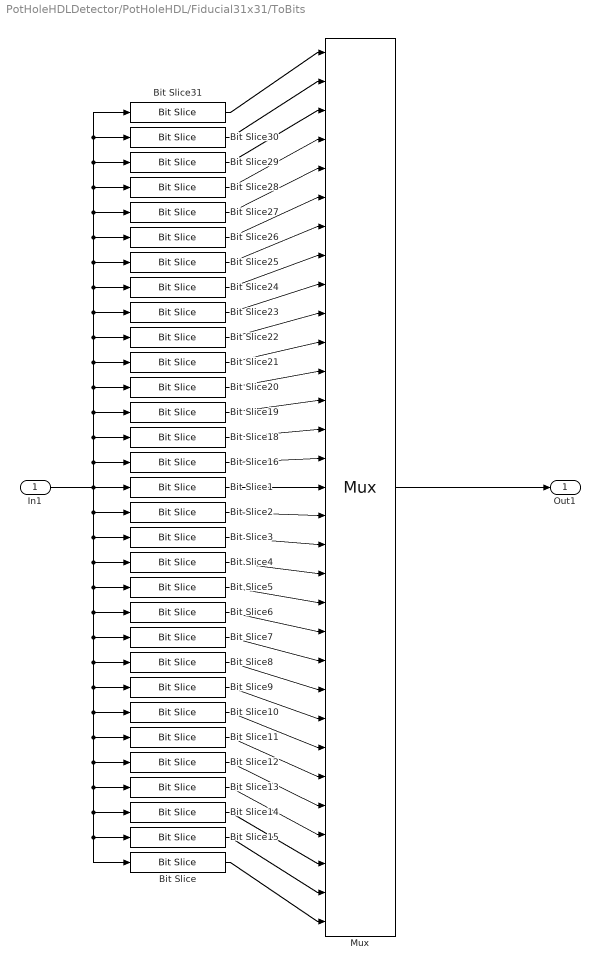
== system PotHoleHDLDetector/PotHoleHDL/Fiducial31x31/ToBits ==
  In1 : Inport
  Bit Slice : hdlsllib/Logic and Bit Operations/Bit Slice  lidx=0  ridx=0
      settings: SourceProductBaseCode=SL
  Bit Slice1 : hdlsllib/Logic and Bit Operations/Bit Slice  lidx=15  ridx=15
      settings: SourceProductBaseCode=SL
  Bit Slice10 : hdlsllib/Logic and Bit Operations/Bit Slice  lidx=6  ridx=6
      settings: SourceProductBaseCode=SL
  Bit Slice11 : hdlsllib/Logic and Bit Operations/Bit Slice  lidx=5  ridx=5
      settings: SourceProductBaseCode=SL
  Bit Slice12 : hdlsllib/Logic and Bit Operations/Bit Slice  lidx=4  ridx=4
      settings: SourceProductBaseCode=SL
  Bit Slice13 : hdlsllib/Logic and Bit Operations/Bit Slice  lidx=3  ridx=3
      settings: SourceProductBaseCode=SL
  Bit Slice14 : hdlsllib/Logic and Bit Operations/Bit Slice  lidx=2  ridx=2
      settings: SourceProductBaseCode=SL
  Bit Slice15 : hdlsllib/Logic and Bit Operations/Bit Slice  lidx=1  ridx=1
      settings: SourceProductBaseCode=SL
  Bit Slice16 : hdlsllib/Logic and Bit Operations/Bit Slice  lidx=16  ridx=16
      settings: SourceProductBaseCode=SL
  Bit Slice18 : hdlsllib/Logic and Bit Operations/Bit Slice  lidx=17  ridx=17
      settings: SourceProductBaseCode=SL
  Bit Slice19 : hdlsllib/Logic and Bit Operations/Bit Slice  lidx=18  ridx=18
      settings: SourceProductBaseCode=SL
  Bit Slice2 : hdlsllib/Logic and Bit Operations/Bit Slice  lidx=14  ridx=14
      settings: SourceProductBaseCode=SL
  Bit Slice20 : hdlsllib/Logic and Bit Operations/Bit Slice  lidx=19  ridx=19
      settings: SourceProductBaseCode=SL
  Bit Slice21 : hdlsllib/Logic and Bit Operations/Bit Slice  lidx=20  ridx=20
      settings: SourceProductBaseCode=SL
  Bit Slice22 : hdlsllib/Logic and Bit Operations/Bit Slice  lidx=21  ridx=21
      settings: SourceProductBaseCode=SL
  Bit Slice23 : hdlsllib/Logic and Bit Operations/Bit Slice  lidx=22  ridx=22
      settings: SourceProductBaseCode=SL
  Bit Slice24 : hdlsllib/Logic and Bit Operations/Bit Slice  lidx=23  ridx=23
      settings: SourceProductBaseCode=SL
  Bit Slice25 : hdlsllib/Logic and Bit Operations/Bit Slice  lidx=24  ridx=24
      settings: SourceProductBaseCode=SL
  Bit Slice26 : hdlsllib/Logic and Bit Operations/Bit Slice  lidx=25  ridx=25
      settings: SourceProductBaseCode=SL
  Bit Slice27 : hdlsllib/Logic and Bit Operations/Bit Slice  lidx=26  ridx=26
      settings: SourceProductBaseCode=SL
  Bit Slice28 : hdlsllib/Logic and Bit Operations/Bit Slice  lidx=27  ridx=27
      settings: SourceProductBaseCode=SL
  Bit Slice29 : hdlsllib/Logic and Bit Operations/Bit Slice  lidx=28  ridx=28
      settings: SourceProductBaseCode=SL
  Bit Slice3 : hdlsllib/Logic and Bit Operations/Bit Slice  lidx=13  ridx=13
      settings: SourceProductBaseCode=SL
  Bit Slice30 : hdlsllib/Logic and Bit Operations/Bit Slice  lidx=29  ridx=29
      settings: SourceProductBaseCode=SL
  Bit Slice31 : hdlsllib/Logic and Bit Operations/Bit Slice  lidx=30  ridx=30
      settings: SourceProductBaseCode=SL
  Bit Slice4 : hdlsllib/Logic and Bit Operations/Bit Slice  lidx=12  ridx=12
      settings: SourceProductBaseCode=SL
  Bit Slice5 : hdlsllib/Logic and Bit Operations/Bit Slice  lidx=11  ridx=11
      settings: SourceProductBaseCode=SL
  Bit Slice6 : hdlsllib/Logic and Bit Operations/Bit Slice  lidx=10  ridx=10
      settings: SourceProductBaseCode=SL
  Bit Slice7 : hdlsllib/Logic and Bit Operations/Bit Slice  lidx=9  ridx=9
      settings: SourceProductBaseCode=SL
  Bit Slice8 : hdlsllib/Logic and Bit Operations/Bit Slice  lidx=8  ridx=8
      settings: SourceProductBaseCode=SL
  Bit Slice9 : hdlsllib/Logic and Bit Operations/Bit Slice  lidx=7  ridx=7
      settings: SourceProductBaseCode=SL
  Mux : Mux  Inputs=31
  Out1 : Outport  VectorParamsAs1DForOutWhenUnconnected=off
  wires:
  In1/1 -> Bit Slice5/1, Bit Slice6/1, Bit Slice7/1, Bit Slice8/1, Bit Slice9/1, Bit Slice10/1, Bit Slice11/1, Bit Slice12/1, Bit Slice13/1, Bit Slice14/1, Bit Slice15/1, Bit Slice/1, Bit Slice4/1, Bit Slice3/1, Bit Slice2/1, Bit Slice16/1, Bit Slice19/1, Bit Slice20/1, Bit Slice21/1, Bit Slice22/1, Bit Slice23/1, Bit Slice24/1, Bit Slice25/1, Bit Slice26/1, Bit Slice27/1, Bit Slice28/1, Bit Slice29/1, Bit Slice30/1, Bit Slice31/1, Bit Slice18/1, Bit Slice1/1
  Mux/1 -> Out1/1
  Bit Slice31/1 -> Mux/1
  Bit Slice30/1 -> Mux/2
  Bit Slice29/1 -> Mux/3
  Bit Slice28/1 -> Mux/4
  Bit Slice27/1 -> Mux/5
  Bit Slice26/1 -> Mux/6
  Bit Slice25/1 -> Mux/7
  Bit Slice24/1 -> Mux/8
  Bit Slice23/1 -> Mux/9
  Bit Slice22/1 -> Mux/10
  Bit Slice21/1 -> Mux/11
  Bit Slice20/1 -> Mux/12
  Bit Slice19/1 -> Mux/13
  Bit Slice18/1 -> Mux/14
  Bit Slice16/1 -> Mux/15
  Bit Slice1/1 -> Mux/16
  Bit Slice2/1 -> Mux/17
  Bit Slice3/1 -> Mux/18
  Bit Slice4/1 -> Mux/19
  Bit Slice5/1 -> Mux/20
  Bit Slice6/1 -> Mux/21
  Bit Slice7/1 -> Mux/22
  Bit Slice8/1 -> Mux/23
  Bit Slice9/1 -> Mux/24
  Bit Slice10/1 -> Mux/25
  Bit Slice11/1 -> Mux/26
  Bit Slice12/1 -> Mux/27
  Bit Slice13/1 -> Mux/28
  Bit Slice14/1 -> Mux/29
  Bit Slice15/1 -> Mux/30
  Bit Slice/1 -> Mux/31

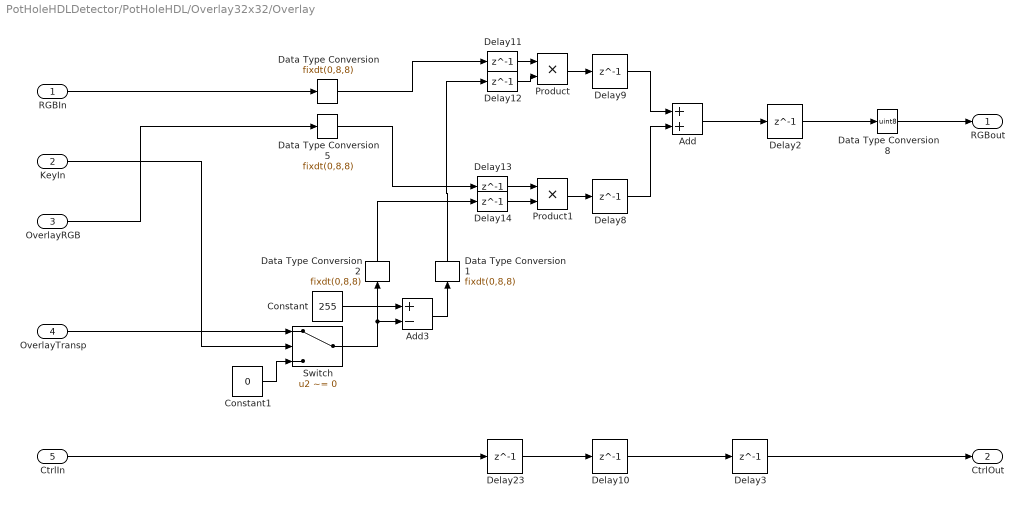
== system PotHoleHDLDetector/PotHoleHDL/Overlay32x32/Overlay ==
  RGBIn : Inport
  KeyIn : Inport  Port=2
  OverlayRGB : Inport  Port=3
  OverlayTransp : Inport  Port=4
  CtrlIn : Inport  Port=5
  Add : Sum  OutDataTypeStr=fixdt(0,8,8)
  Add3 : Sum  Inputs=+-  OutDataTypeStr=uint8
  Constant : Constant  Value=255  OutDataTypeStr=uint8  SampleTime=-1
  Constant1 : Constant  Value=0  OutDataTypeStr=uint8
  Data Type Conversion{,1..2,5} (4 alike) : DataTypeConversion  OutDataTypeStr=fixdt(0,8,8)  ConvertRealWorld=Stored Integer (SI)  SaturateOnIntegerOverflow=off  RndMeth=Floor
  Data Type Conversion8 : DataTypeConversion  OutDataTypeStr=uint8  ConvertRealWorld=Stored Integer (SI)  SaturateOnIntegerOverflow=off  RndMeth=Floor
  Delay{2..3,8..14,23} (10 alike) : Delay  DelayLength=1
  Product : Product  OutDataTypeStr=fixdt(0,8,8)  SaturateOnIntegerOverflow=on
  Product1 : Product  OutDataTypeStr=fixdt(0,8,8)  SaturateOnIntegerOverflow=on
  Switch : Switch  Criteria=u2 ~= 0  SaturateOnIntegerOverflow=off  InputSameDT=off
  RGBout : Outport  VectorParamsAs1DForOutWhenUnconnected=off
  "CtrlOut " : Outport  Port=2  VectorParamsAs1DForOutWhenUnconnected=off
  wires:
  Add/1 -> Delay2/1
  Constant/1 -> Add3/1
  Add3/1 -> Data Type Conversion1/1
  Switch/1 -> Data Type Conversion2/1, Add3/2
  OverlayTransp/1 -> Switch/1
  KeyIn/1 -> Switch/2
  Constant1/1 -> Switch/3
  Delay2/1 -> Data Type Conversion8/1
  Delay3/1 -> "CtrlOut "/1
  Product1/1 -> Delay8/1
  Product/1 -> Delay9/1
  Delay9/1 -> Add/1
  Delay8/1 -> Add/2
  Delay10/1 -> Delay3/1
  Delay11/1 -> Product/1
  Delay12/1 -> Product/2
  Delay13/1 -> Product1/1
  Delay14/1 -> Product1/2
  Delay23/1 -> Delay10/1
  CtrlIn/1 -> Delay23/1
  Data Type Conversion/1 -> Delay11/1
  Data Type Conversion1/1 -> Delay12/1
  Data Type Conversion2/1 -> Delay14/1
  OverlayRGB/1 -> Data Type Conversion5/1
  RGBIn/1 -> Data Type Conversion/1
  Data Type Conversion8/1 -> RGBout/1
  Data Type Conversion5/1 -> Delay13/1

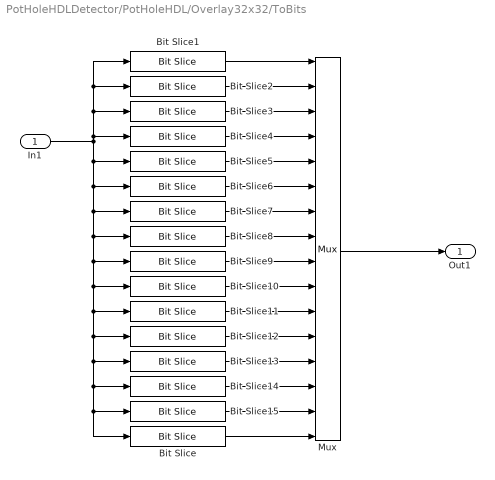
== system PotHoleHDLDetector/PotHoleHDL/Overlay32x32/ToBits ==
  In1 : Inport
  Bit Slice : hdlsllib/Logic and Bit Operations/Bit Slice  lidx=0  ridx=0
      settings: SourceProductBaseCode=SL
  Bit Slice1 : hdlsllib/Logic and Bit Operations/Bit Slice  lidx=15  ridx=15
      settings: SourceProductBaseCode=SL
  Bit Slice10 : hdlsllib/Logic and Bit Operations/Bit Slice  lidx=6  ridx=6
      settings: SourceProductBaseCode=SL
  Bit Slice11 : hdlsllib/Logic and Bit Operations/Bit Slice  lidx=5  ridx=5
      settings: SourceProductBaseCode=SL
  Bit Slice12 : hdlsllib/Logic and Bit Operations/Bit Slice  lidx=4  ridx=4
      settings: SourceProductBaseCode=SL
  Bit Slice13 : hdlsllib/Logic and Bit Operations/Bit Slice  lidx=3  ridx=3
      settings: SourceProductBaseCode=SL
  Bit Slice14 : hdlsllib/Logic and Bit Operations/Bit Slice  lidx=2  ridx=2
      settings: SourceProductBaseCode=SL
  Bit Slice15 : hdlsllib/Logic and Bit Operations/Bit Slice  lidx=1  ridx=1
      settings: SourceProductBaseCode=SL
  Bit Slice2 : hdlsllib/Logic and Bit Operations/Bit Slice  lidx=14  ridx=14
      settings: SourceProductBaseCode=SL
  Bit Slice3 : hdlsllib/Logic and Bit Operations/Bit Slice  lidx=13  ridx=13
      settings: SourceProductBaseCode=SL
  Bit Slice4 : hdlsllib/Logic and Bit Operations/Bit Slice  lidx=12  ridx=12
      settings: SourceProductBaseCode=SL
  Bit Slice5 : hdlsllib/Logic and Bit Operations/Bit Slice  lidx=11  ridx=11
      settings: SourceProductBaseCode=SL
  Bit Slice6 : hdlsllib/Logic and Bit Operations/Bit Slice  lidx=10  ridx=10
      settings: SourceProductBaseCode=SL
  Bit Slice7 : hdlsllib/Logic and Bit Operations/Bit Slice  lidx=9  ridx=9
      settings: SourceProductBaseCode=SL
  Bit Slice8 : hdlsllib/Logic and Bit Operations/Bit Slice  lidx=8  ridx=8
      settings: SourceProductBaseCode=SL
  Bit Slice9 : hdlsllib/Logic and Bit Operations/Bit Slice  lidx=7  ridx=7
      settings: SourceProductBaseCode=SL
  Mux : Mux  Inputs=16
  Out1 : Outport  VectorParamsAs1DForOutWhenUnconnected=off
  wires:
  In1/1 -> Bit Slice5/1, Bit Slice6/1, Bit Slice7/1, Bit Slice8/1, Bit Slice9/1, Bit Slice10/1, Bit Slice11/1, Bit Slice12/1, Bit Slice13/1, Bit Slice14/1, Bit Slice15/1, Bit Slice/1, Bit Slice4/1, Bit Slice3/1, Bit Slice2/1, Bit Slice1/1
  Bit Slice7/1 -> Mux/7
  Bit Slice8/1 -> Mux/8
  Bit Slice9/1 -> Mux/9
  Bit Slice13/1 -> Mux/13
  Bit Slice6/1 -> Mux/6
  Bit Slice4/1 -> Mux/4
  Bit Slice2/1 -> Mux/2
  Bit Slice/1 -> Mux/16
  Mux/1 -> Out1/1
  Bit Slice15/1 -> Mux/15
  Bit Slice11/1 -> Mux/11
  Bit Slice5/1 -> Mux/5
  Bit Slice1/1 -> Mux/1
  Bit Slice12/1 -> Mux/12
  Bit Slice3/1 -> Mux/3
  Bit Slice14/1 -> Mux/14
  Bit Slice10/1 -> Mux/10

== system PotHoleHDLDetector/PotHoleHDL/Centroid31/CentroidKernel/EnTapDelay23 ==
  In1 : Inport
  Enable : EnablePort
  State Control : StateControl  StateControl=Synchronous
  Tapped Delay : simulink/Discrete/Tapped Delay  vinit=0.0  samptime=-1  NumDelays=31  DelayOrder=Oldest  includeCurrent=off
  Out1 : Outport  VectorParamsAs1DForOutWhenUnconnected=off
  wires:
  Tapped Delay/1 -> Out1/1
  In1/1 -> Tapped Delay/1

== system PotHoleHDLDetector/PotHoleHDL/Centroid31/CentroidKernel/EnTapDelay32 ==
  In1 : Inport
  Enable : EnablePort
  State Control : StateControl  StateControl=Synchronous
  Tapped Delay : simulink/Discrete/Tapped Delay  vinit=0.0  samptime=-1  NumDelays=31  DelayOrder=Oldest  includeCurrent=off
  Out1 : Outport  VectorParamsAs1DForOutWhenUnconnected=off
  wires:
  In1/1 -> Tapped Delay/1
  Tapped Delay/1 -> Out1/1
